simulink model "EjemploSMC_seg_tray_forma1"  (R2026b)
settings: Solver=ode4  StopTime=20  FixedStep=0.0001
settings Model: Creator=nestorhernandezcastellanos  LastModifiedBy=nestorhernandezcastellanos

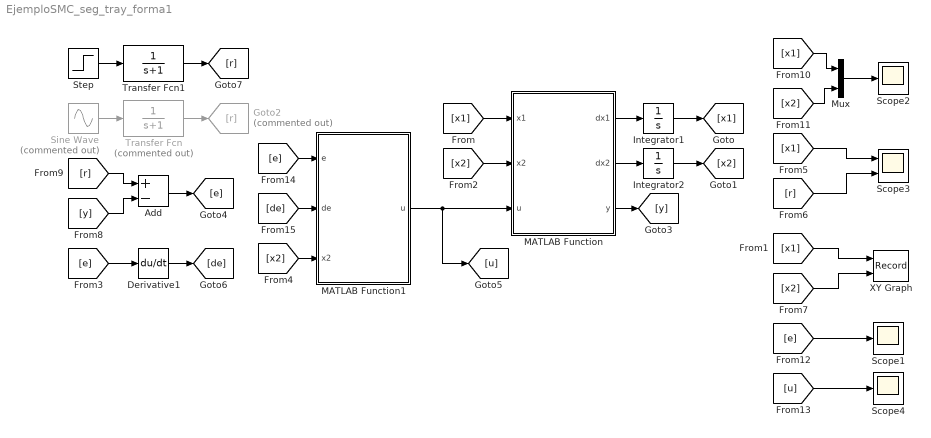
== system EjemploSMC_seg_tray_forma1 ==
  Add : Sum  Inputs=+-
  Derivative1 : Derivative
  Goto2 : Goto  Commented=on  GotoTag=r
  Integrator1 : Integrator  InitialCondition=1
  Integrator2 : Integrator  InitialCondition=-2
  MATLAB Function : MATLAB Function  TreatAsAtomicUnit=on
  MATLAB Function1 : MATLAB Function  TreatAsAtomicUnit=on
  Mux : Mux  Inputs=2
  Scope1 : Scope
      settings: ActiveDisplayYMinimum=-1.1250001628551478  ActiveDisplayYMaximum=0.12500146569633067
  Scope2 : Scope
      settings: ActiveDisplayYMinimum=-2.3780113002128531  ActiveDisplayYMaximum=1.4021017019156774  DataLoggingVariableName=ScopeData2
  Scope3 : Scope  NumInputPorts=2
      settings: ActiveDisplayYMinimum=-0.12500685330295525  ActiveDisplayYMaximum=1.1250616797265975  DataLoggingVariableName=ScopeData3
  Scope4 : Scope
      settings: ActiveDisplayYMinimum=-6.5000137349379781  ActiveDisplayYMaximum=8.498947657870163
  Sine Wave : Sin  Commented=on  SampleTime=0
  Step : Step  SampleTime=0
  Transfer Fcn : TransferFcn  Commented=on  Denominator=[1 1]
  Transfer Fcn1 : TransferFcn  Denominator=[1 1]
  XY Graph : Record  NumPorts=2.0  FileSettingsInternal="{\"entries\":[{\"content\":{\"excelSettings\":{\"content\":{},\"type\":\"Streamout.ExcelSettings\"},\"parquetSettings\":{\"content\":{},\"type\":\"Streamout.ParquetSettings\"}},\"type\":\"Streamout.FileSettingStorage\",\"uuid\":\"\"}],\"packageUris\":[\"http:\\/\\/schema.mathworks.com\\/mf0\\/streamout_blocks\\/R2020a\"],\"version\":\"1.0\"}"  FrameSettings=[0, 0]  Layout=[1 1]  SignalsInternal="{\"entries\":[{\"content\":{\"signals\":[{\"content\":{\"blockPath\":[],\"dimensions\":[1],\"domain\":\"\",\"lineColor\":\"#a2142f\",\"plots\":[ 1 ],\"port\":1,\"sid\":[\"\"],\"signalID\":1,\"signalName\":\"From1\"},\"type\":\"RecordBlkView.Signal\",\"uuid\":\"\"},{\"content\":{\"blockPath\":[],\"dimensions\":[1],\"domain\":\"\",\"lineColor\":\"#139fff\",\"plots\":[ 1 ],\"port\":2,\"sid\":[\"\"],\"signalID\":2,\"signalName\":\"From7\"},\"type\":\"RecordBlkView.Signal\",\"uuid\":\"\"}]},\"type\":\"RecordBlkView.InputSignals\",\"uuid\":\"\"}],\"packageUris\":[\"http:\\/\\/schema.mathworks.com\\/mf0\\/streamout_blocks\\/R2020a\"],\"version\":\"1.0\"}"  VisualizationBindings="{\"xyplotplugin\":{\"info\":[{\"series\":[{\"bindingParametersList\":[{\"parameter\":\"X-Axis\",\"signalID\":1,\"signalName\":\"From1\"},{\"parameter\":\"Y-Axis\",\"signalID\":2,\"signalName\":\"From7\"}],\"seriesID\":0}],\"subplotID\":1}]}}"  CompatibilityTag=XY
  wires:
  MATLAB Function1/1(u) -> [u], MATLAB Function/3(u)
  MATLAB Function/2(dx2) -> Integrator2/1
  MATLAB Function/1(dx1) -> Integrator1/1
  Mux/1 -> Scope2/1
  Sine Wave/1 -> Transfer Fcn/1
  [x1] -> MATLAB Function/1(x1)
  [x1] -> XY Graph/1
  [x2] -> MATLAB Function/2(x2)
  [x2] -> MATLAB Function1/3(x2)
  [x1] -> Scope3/1
  [r] -> Scope3/2
  [x2] -> XY Graph/2
  Integrator2/1 -> [x2]
  Integrator1/1 -> [x1]
  MATLAB Function/3(y) -> [y]
  [y] -> Add/2
  [r] -> Add/1
  [x2] -> Mux/2
  [x1] -> Mux/1
  [e] -> Scope1/1
  [u] -> Scope4/1
  Add/1 -> [e]
  [e] -> MATLAB Function1/1(e)
  [e] -> Derivative1/1
  Derivative1/1 -> [de]
  [de] -> MATLAB Function1/2(de)
  Transfer Fcn/1 -> Goto2/1
  Transfer Fcn1/1 -> [r]
  Step/1 -> Transfer Fcn1/1

== matlab function EjemploSMC_seg_tray_forma1/MATLAB Function1 ==
  data: e input; de input; x2 input; u output
function u = controlador(e, de, x2)

% Ganancia K>2
K = 3;

% Valor arbitrario positivo
m = 2;

sigma = de + m*e;
u = -m*x2 + K*sign(sigma);

== matlab function EjemploSMC_seg_tray_forma1/MATLAB Function ==
  data: x1 input; x2 input; dx1 output; u input; dx2 output; y output
function [dx1, dx2, y] = planta(x1, x2, u)

dx1 = x2;
dx2 = sin(x1+x2) + cos(x1*x2) + u;

y = x1;
